simulink model "prob2markov"  (R2019a)
settings: Solver=VariableStepAuto  StartTime=0.0  StopTime=10.0  RelTol=1e-3
values from neighbouring files (symbols this model uses):
  bias = 1E-3 * g    [prob2main.m]
  C1 = 2 / tau    [prob2main.m]
  C2 = 1/tau/tau + 2 * schuler^2    [prob2main.m]
  schuler = sqrt(g/R)    [prob2main.m]
undefined symbols (not defined in the file or in its folder): tauH, varH
settings Model: Creator=hyunwoong  LastModifiedBy=hyunwoong

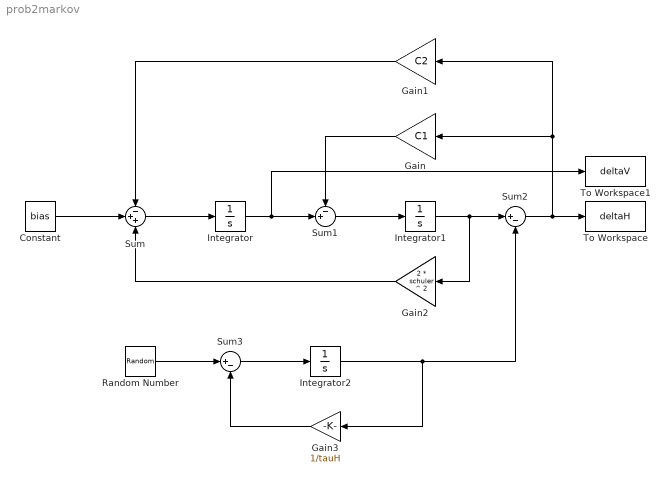
== system prob2markov ==
  Constant : Constant  Value=bias
  Gain : Gain  Gain=C1
  Gain1 : Gain  Gain=C2
  Gain2 : Gain  Gain=2 * schuler ^ 2
  Gain3 : Gain  Gain=1/tauH
  Integrator : Integrator
  Integrator1 : Integrator
  Integrator2 : Integrator
  Random Number : RandomNumber  Variance=varH  SampleTime=0.005
  Sum : Sum  Inputs=-++
  Sum1 : Sum  Inputs=-+|
  Sum2 : Sum  Inputs=|+-
  Sum3 : Sum  Inputs=|+-
  To Workspace : ToWorkspace  VariableName=deltaH  SaveFormat=Timeseries  SampleTime=-1
  To Workspace1 : ToWorkspace  VariableName=deltaV  SaveFormat=Timeseries  SampleTime=-1
  wires:
  Sum/1 -> Integrator/1
  Integrator/1 -> To Workspace1/1, Sum1/2
  Sum1/1 -> Integrator1/1
  Integrator1/1 -> Sum2/1, Gain2/1
  Sum2/1 -> To Workspace/1, Gain1/1, Gain/1
  Gain/1 -> Sum1/1
  Gain1/1 -> Sum/1
  Gain2/1 -> Sum/3
  Sum3/1 -> Integrator2/1
  Integrator2/1 -> Gain3/1, Sum2/2
  Gain3/1 -> Sum3/2
  Random Number/1 -> Sum3/1
  Constant/1 -> Sum/2
